simulink library "SUB_PLANT_Chassis"  (R2018a)
settings: Solver=VariableStepAuto  StartTime=0.0  StopTime=10.0  RelTol=1e-3
values from neighbouring files (symbols this model uses):
  Cf = 120000    [SUB_PLANT_LateralDynamics_CAL.mat]
  Cr = 240000    [SUB_PLANT_LateralDynamics_CAL.mat]
  GLB_FIXED_STEP_SIZE_CPV = ptc_matlab_lib.PTC_MBDS_Parameter('Value', 0.01,  	'Description', 'Global Fixed Step Size (Fundamental Sample Time)',  	'Unit', 's',  	'CoderInfo.StorageClass', 'Custom',  	'CoderInfo.CustomStorageClass', 'Const')    [GLB_CONST.m]
  heading_0 = 5.2    [SUB_PLANT_LateralDynamics_CAL.mat]
  Iz = 10000    [SUB_PLANT_LateralDynamics_CAL.mat]
  lf = 2.5    [SUB_PLANT_LateralDynamics_CAL.mat]
  lr = 3.5    [SUB_PLANT_LateralDynamics_CAL.mat]
  Vx_0 = 1    [SUB_PLANT_LateralDynamics_CAL.mat]
undefined symbols (not defined in the file or in its folder): DiscIntNeverNeededParam, GLB_TRANS_LOSS_TRQ_GEAR_STEP_MPV, GLB_TRANS_LOSS_TRQ_SPD_STEP_MPV, GLB_TRANS_LOSS_TRQ_TABLE_DATA_MPV, GLB_TRANS_LOSS_TRQ_TRQ_STEP_MPV
libraries: PTC_MBDS_LIB x41, simulink x6
(part 1 of 2)
settings Model: Creator=Sundeep.Tuteja  LastModifiedBy=Haris.Ashraf

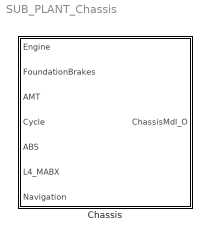
== system SUB_PLANT_Chassis ==
  Chassis : Subsystem

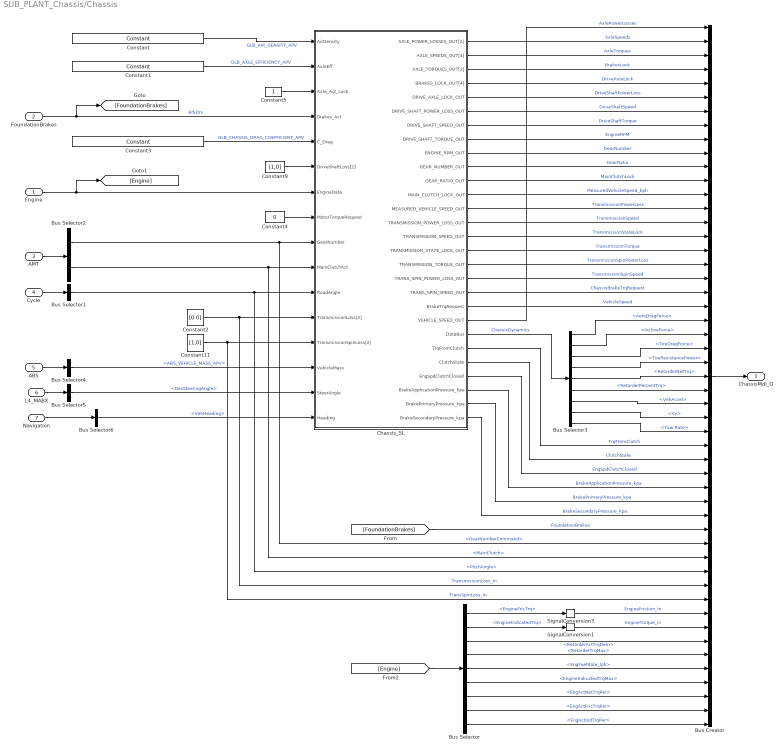
== system SUB_PLANT_Chassis/Chassis ==
  Engine : Inport
  FoundationBrakes : Inport  Port=2
  AMT : Inport  Port=3
  Cycle : Inport  Port=4
  ABS : Inport  Port=5
  L4_MABX : Inport  Port=6
  Navigation : Inport  Port=7
  Bus Creator : BusCreator  Inputs=51
  Bus Selector : BusSelector  OutputSignals=EngineFricTrq,EngineIndicatedTrq,RetarderActTrqDem,RetarderTrqMax,EngFuelRate_lph,EngineIndicatedTrqMax,EngActNetTrqPer,EngActFricTrqPer,EngActIndTrqPer
  Bus Selector1 : BusSelector  OutputSignals=PitchAngle
  Bus Selector2 : BusSelector  OutputSignals=ShiftControl.Internal.GearNumberCommand,ShiftControl.Internal.MainClutch
  Bus Selector3 : BusSelector  OutputSignals=AeroDragForce,InclineForce,TireDragForce,TireResistancePower,RetarderNetTrq,RetarderPercentTrq,VehAccel,Vy,Yaw Rate
  Bus Selector4 : BusSelector  OutputSignals=ABS_VEHICLE_MASS_APV
  Bus Selector5 : BusSelector  OutputSignals=10msTask.SteeringControl.DesSteeringAngle
  Bus Selector6 : BusSelector  OutputSignals=Navigation.VehHeading
  Chassis_SL : Subsystem
  Constant : PTC_MBDS_LIB/Extras/Sources/Constant  Value2=GLB_AIR_DENSITY_APV  PTC_MBDS_BlockVersion=5.41  PTC_BlockType=PTC_MBDS_Constant
      settings: SourceProductName=PACCAR Technical Center MBDS Library
      settings: AttributesFormatString=|
      | Value: 1.23696005344
      | Unit: 'kg/m^3'
  Constant1 : PTC_MBDS_LIB/Extras/Sources/Constant  Value2=GLB_AXLE_EFFICIENCY_APV  PTC_MBDS_BlockVersion=5.41  PTC_BlockType=PTC_MBDS_Constant
      settings: SourceProductName=PACCAR Technical Center MBDS Library
      settings: AttributesFormatString=|
      | Value: 0.980000019073
      | Unit: '1'
  Constant11 : Constant  Value=[1,0]
  Constant2 : Constant  Value=[0 0]
  Constant3 : PTC_MBDS_LIB/Extras/Sources/Constant  Value2=GLB_CHASSIS_DRAG_COEFFICIENT_APV  PTC_MBDS_BlockVersion=5.41  PTC_BlockType=PTC_MBDS_Constant
      settings: SourceProductName=PACCAR Technical Center MBDS Library
      settings: AttributesFormatString=|
      | Value: 0.65
      | Unit: '1'
  Constant4 : Constant  Value=0
  Constant5 : Constant
  Constant9 : Constant  Value=[1,0]
  SignalConversion1 : SignalConversion  ConversionOutput=Contiguous copy  OverrideOpt=off
  SignalConversion3 : SignalConversion  ConversionOutput=Contiguous copy  OverrideOpt=off
  ChassisMdl_O : Outport
  wires:
  Bus Selector6/1 -> Chassis_SL/16(Heading)  "<VehHeading>"
  Navigation/1 -> Bus Selector6/1
  Chassis_SL/25(EngSpdClutchClosed) -> Bus Creator/33  "EngSpdClutchClosed"
  Chassis_SL/24(ClutchState) -> Bus Creator/32  "ClutchState"
  Chassis_SL/23(TrqFromClutch) -> Bus Creator/31  "TrqFromClutch"
  Bus Selector2/1 -> Chassis_SL/9(GearNumber), Bus Creator/38  "<GearNumberCommand>"
  Chassis_SL/5(DRIVE_AXLE_LOCK_OUT) -> Bus Creator/5  "DriveAxleLock"
  Chassis_SL/11(GEAR_RATIO_OUT) -> Bus Creator/11  "GearRatio"
  Chassis_SL/3(AXLE_TORQUES_OUT[2]) -> Bus Creator/3  "AxleTorques"
  Chassis_SL/19(TRANS_SPIN_SPEED_OUT) -> Bus Creator/19  "TransmissionSpinSpeed"
  Chassis_SL/7(DRIVE_SHAFT_SPEED_OUT) -> Bus Creator/7  "DriveShaftSpeed"
  Chassis_SL/4(BRAKES_LOCK_OUT[4]) -> Bus Creator/4  "BrakesLock"
  Chassis_SL/18(TRANS_SPIN_POWER_LOSS_OUT) -> Bus Creator/18  "TransmissionSpinPowerLoss"
  Chassis_SL/6(DRIVE_SHAFT_POWER_LOSS_OUT) -> Bus Creator/6  "DrIveShaftPowerLoss"
  Chassis_SL/20(BrakeTrqRequest) -> Bus Creator/20  "ChassisBrakeTrqRequest"
  Chassis_SL/8(DRIVE_SHAFT_TORQUE_OUT) -> Bus Creator/8  "DriveShaftTorque"
  Chassis_SL/14(TRANSMISSION_POWER_LOSS_OUT) -> Bus Creator/14  "TransmissionPowerLoss"
  Constant1/1 -> Chassis_SL/2(AxleEff)  "GLB_AXLE_EFFICIENCY_APV"
  Constant5/1 -> Chassis_SL/3(Axle_Act_Lock)
  Constant3/1 -> Chassis_SL/5(C_Drag)  "GLB_CHASSIS_DRAG_COEFFICIENT_APV"
  Constant9/1 -> Chassis_SL/6(DriveShaftLoss[2])
  Constant11/1 -> Chassis_SL/13(TransmissionSpinLoss[2]), Bus Creator/42  "TransSpinLoss_In"
  Constant2/1 -> Chassis_SL/12(TransmissionLoss[2]), Bus Creator/41  "TransmisisonLoss_In"
  Bus Selector2/2 -> Bus Creator/39, Chassis_SL/10(MainClutchAct)  "<MainClutch>"
  Bus Creator/1 -> ChassisMdl_O/1
  Chassis_SL/1(AXLE_POWER_LOSSES_OUT[2]) -> Bus Creator/1  "AxlePowerLosses"
  Chassis_SL/9(ENGINE_RPM_OUT) -> Bus Creator/9  "EngineRPM"
  Chassis_SL/10(GEAR_NUMBER_OUT) -> Bus Creator/10  "GearNumber"
  Chassis_SL/12(MAIN_CLUTCH_LOCK_OUT) -> Bus Creator/12  "MainClutchLock"
  Chassis_SL/13(MEASURED_VEHICLE_SPEED_OUT) -> Bus Creator/13  "MeasuredVehicleSpeed_kph"
  Chassis_SL/16(TRANSMISSION_STATE_LOCK_OUT) -> Bus Creator/16  "TransmissionStateLock"
  Chassis_SL/17(TRANSMISSION_TORQUE_OUT) -> Bus Creator/17  "TransmissionTorque"
  Cycle/1 -> Bus Selector1/1
  Bus Selector1/1 -> Bus Creator/40, Chassis_SL/11(RoadAngle)  "<PitchAngle>"
  AMT/1 -> Bus Selector2/1
  FoundationBrakes/1 -> [FoundationBrakes], Chassis_SL/4(Brakes_Act)  "BrkDrv"
  [FoundationBrakes] -> Bus Creator/37  "FoundationBrakes"
  Bus Selector/7 -> Bus Creator/49  "<EngActNetTrqPer>"
  Bus Selector/8 -> Bus Creator/50  "<EngActFricTrqPer>"
  Chassis_SL/2(AXLE_SPEEDS_OUT[4]) -> Bus Creator/2  "AxleSpeeds"
  Chassis_SL/22(DataBus) -> Bus Selector3/1  "ChassisDynamics"
  Bus Selector3/1 -> Bus Creator/22  "<AeroDragForce>"
  Bus Selector3/2 -> Bus Creator/23  "<InclineForce>"
  Bus Selector3/4 -> Bus Creator/25  "<TireResistancePower>"
  Bus Selector3/5 -> Bus Creator/26  "<RetarderNetTrq>"
  Engine/1 -> [Engine], Chassis_SL/7(EngineData)
  [Engine] -> Bus Selector/1
  Bus Selector/1 -> SignalConversion3/1  "<EngineFricTrq>"
  Bus Selector/2 -> SignalConversion1/1  "<EngineIndicatedTrq>"
  Bus Selector3/6 -> Bus Creator/27  "<RetarderPercentTrq>"
  Bus Selector/3 -> Bus Creator/45  "<RetarderActTrqDem>"
  Bus Selector/4 -> Bus Creator/46  "<RetarderTrqMax>"
  Bus Selector3/7 -> Bus Creator/28  "<VehAccel>"
  Bus Selector/5 -> Bus Creator/47  "<EngFuelRate_lph>"
  Bus Selector3/3 -> Bus Creator/24  "<TireDragForce>"
  Bus Selector/6 -> Bus Creator/48  "<EngineIndicatedTrqMax>"
  Constant/1 -> Chassis_SL/1(AirDensity)  "GLB_AIR_DENSITY_APV"
  ABS/1 -> Bus Selector4/1
  Bus Selector4/1 -> Chassis_SL/14(VehicleMass)  "<ABS_VEHICLE_MASS_APV>"
  Chassis_SL/15(TRANSMISSION_SPEED_OUT) -> Bus Creator/15  "TransmissionSpeed"
  Chassis_SL/21(VEHICLE_SPEED_OUT) -> Bus Creator/21  "VehicleSpeed"
  Bus Selector/9 -> Bus Creator/51  "<EngActIndTrqPer>"
  SignalConversion3/1 -> Bus Creator/43  "EngineFriction_In"
  SignalConversion1/1 -> Bus Creator/44  "EngineTorque_in"
  Constant4/1 -> Chassis_SL/8(MotorTorqueRequest)
  Chassis_SL/26(BrakeApplicationPressure_kpa) -> Bus Creator/34  "BrakeApplicationPressure_kpa"
  Chassis_SL/27(BrakePrimaryPressure_kpa) -> Bus Creator/35  "BrakePrimaryPressure_kpa"
  Chassis_SL/28(BrakeSecondaryPressure_kpa) -> Bus Creator/36  "BrakeSecondaryPressure_kpa"
  Bus Selector3/8 -> Bus Creator/29  "<Vy>"
  Bus Selector3/9 -> Bus Creator/30  "<Yaw Rate>"
  L4_MABX/1 -> Bus Selector5/1
  Bus Selector5/1 -> Chassis_SL/15(SteerAngle)  "<DesSteeringAngle>"

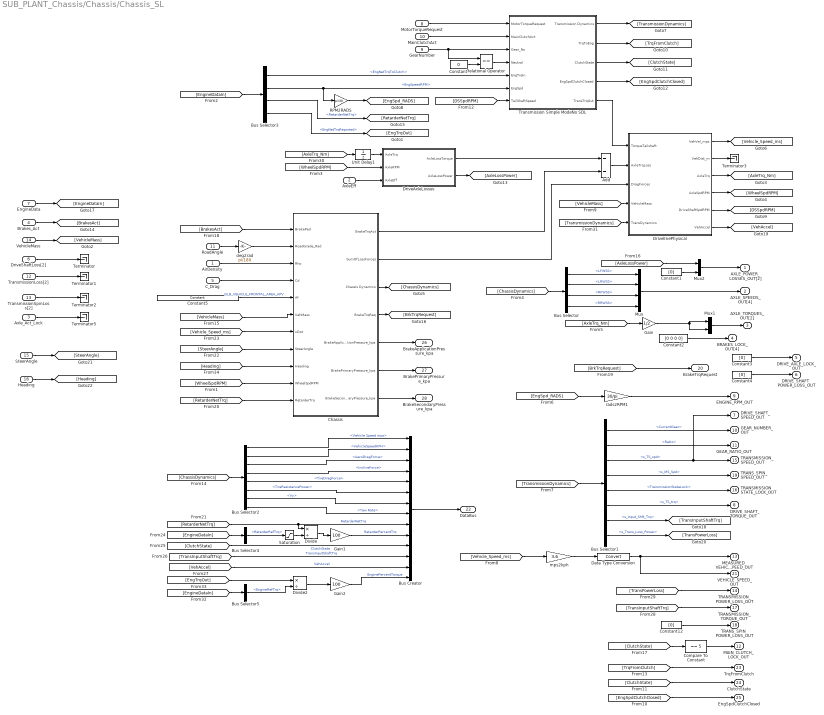
== system SUB_PLANT_Chassis/Chassis/Chassis_SL ==
  AirDensity : Inport
  AxleEff : Inport  Port=2
  Axle_Act_Lock : Inport  Port=3
  Brakes_Act : Inport  Port=4
  C_Drag : Inport  Port=5
  DriveShaftLoss[2] : Inport  Port=6
  EngineData : Inport  Port=7
  MotorTorqueRequest : Inport  Port=8
  GearNumber : Inport  Port=9
  MainClutchAct : Inport  Port=10
  RoadAngle : Inport  Port=11
  TransmissionLoss[2] : Inport  Port=12
  TransmissionSpinLoss[2] : Inport  Port=13
  VehicleMass : Inport  Port=14
  SteerAngle : Inport  Port=15
  Heading : Inport  Port=16
  Add : Sum  Inputs=--
  Bus Creator : BusCreator  Inputs=14
  Bus Selector : BusSelector  OutputSignals=Wheel Speed Sensors.LFWSS,Wheel Speed Sensors.LRWSS,Wheel Speed Sensors.RFWSS,Wheel Speed Sensors.RRWSS
  Bus Selector1 : BusSelector  OutputSignals=Gears_bus.CurrentGear,Gears_bus.Ratio,Gears_bus.s_TS_spd,Gears_bus.s_MS_Spd,MainClutch_bus.TransmissionStateLock,Gears_bus.s_TS_trq,s_Input_Shft_Trq,Gears_bus.s_Trans_Loss_Power
  Bus Selector2 : BusSelector  OutputSignals=Vehicle Speed mps,VehicleSpeedKPH,LongitudnalDynamics.AeroDragForce,LongitudnalDynamics.InclineForce,LongitudnalDynamics.TireDragForce,TireResistancePower,LateralDynamics.Vy,LateralDynamics.Yaw Rate
  Bus Selector3 : BusSelector  OutputSignals=EngNetTrqToClutch,EngSpeedRPM,RetarderNetTrq,EngNetTrqReported
  Bus Selector4 : BusSelector  OutputSignals=RetarderRefTrq
  Bus Selector5 : BusSelector  OutputSignals=EngineRefTrq
  Chassis : Subsystem
  Compare To Constant : simulink/Logic and Bit Operations/Compare To Constant  relop===  const=5  OutDataTypeStr=boolean
  Constant : Constant  Value=0
  Constant{1,3..4,12} (4 alike) : Constant  Value=[0]
  Constant2 : Constant  Value=[0 0 0 0]
  Constant5 : PTC_MBDS_LIB/Extras/Sources/Constant  Value2=GLB_VEHICLE_FRONTAL_AREA_APV  PTC_MBDS_BlockVersion=5.41  PTC_BlockType=PTC_MBDS_Constant
      settings: SourceProductName=PACCAR Technical Center MBDS Library
      settings: AttributesFormatString=|
      | Value: 10.38
      | Unit: 'm^2'
  Data Type Conversion : DataTypeConversion  SaturateOnIntegerOverflow=on
  Divide : Product  Inputs=*/
  Divide2 : Product  Inputs=*/
  DriveAxleLosses : Subsystem
  DrivelInePhysical : Subsystem
  Gain : Gain  Gain=1/2
  Gain1 : Gain  Gain=100
  Gain2 : Gain  Gain=100
  Mux : Mux
  Mux1 : Mux  Inputs=2
  Mux2 : Mux  Inputs=2
  RPM2RADS : Gain  Gain=pi/30
  Relational Operator : RelationalOperator  Operator===  OutDataTypeStr=boolean  RndMeth=Nearest
  Saturation : Saturate  UpperLimit=inf  LowerLimit=1
  Terminator{,1..3,5} (5 alike) : Terminator
      Terminator3 settings: InitFcn=|
      | try
      |    MBDS_BlockCallback('Update', gcb);
      | end
  Transmission Simple ModeNo SDL : Subsystem
  Unit Delay1 : UnitDelay  SampleTime=-1
  deg2rad : Gain  Gain=pi/180
  mps2kph : Gain  Gain=3.6
  rads2RPM1 : Gain  Gain=30/pi
  AXLE_POWER_LOSSES_OUT[2] : Outport
  AXLE_SPEEDS_OUT[4] : Outport  Port=2
  AXLE_TORQUES_OUT[2] : Outport  Port=3
  BRAKES_LOCK_OUT[4] : Outport  Port=4
  DRIVE_AXLE_LOCK_OUT : Outport  Port=5
  DRIVE_SHAFT_POWER_LOSS_OUT : Outport  Port=6
  DRIVE_SHAFT_SPEED_OUT : Outport  Port=7
  DRIVE_SHAFT_TORQUE_OUT : Outport  Port=8
  ENGINE_RPM_OUT : Outport  Port=9
  GEAR_NUMBER_OUT : Outport  Port=10
  GEAR_RATIO_OUT : Outport  Port=11
  MAIN_CLUTCH_LOCK_OUT : Outport  Port=12
  MEASURED_VEHICLE_SPEED_OUT : Outport  Port=13
  TRANSMISSION_POWER_LOSS_OUT : Outport  Port=14
  TRANSMISSION_SPEED_OUT : Outport  Port=15
  TRANSMISSION_STATE_LOCK_OUT : Outport  Port=16
  TRANSMISSION_TORQUE_OUT : Outport  Port=17
  TRANS_SPIN_POWER_LOSS_OUT : Outport  Port=18
  TRANS_SPIN_SPEED_OUT : Outport  Port=19
  BrakeTrqRequest : Outport  Port=20
  VEHICLE_SPEED_OUT : Outport  Port=21
  DataBus : Outport  Port=22
  TrqFromClutch : Outport  Port=23
  ClutchState : Outport  Port=24
  EngSpdClutchClosed : Outport  Port=25
  BrakeApplicationPressure_kpa : Outport  Port=26
  BrakePrimaryPressure_kpa : Outport  Port=27
  BrakeSecondaryPressure_kpa : Outport  Port=28
  wires:
  MotorTorqueRequest/1 -> Transmission Simple ModeNo SDL/1(MotorTorqueRequest)
  Bus Selector3/3 -> [RetarderNetTrq]  "<RetarderNetTrq>"
  Bus Selector3/2 -> Transmission Simple ModeNo SDL/6(EngSpd), RPM2RADS/1  "<EngSpeedRPM>"
  [EngineDataIn] -> Bus Selector3/1
  AirDensity/1 -> Chassis/3(Rho)
  C_Drag/1 -> Chassis/4(Cd)
  Constant5/1 -> Chassis/5(Af)  "GLB_VEHICLE_FRONTAL_AREA_APV"
  RoadAngle/1 -> deg2rad/1
  deg2rad/1 -> Chassis/2(RoadGrade_Rad)
  MainClutchAct/1 -> Transmission Simple ModeNo SDL/2(MainClutchAct)
  GearNumber/1 -> Relational Operator/1, Transmission Simple ModeNo SDL/3(Gear_No)
  Relational Operator/1 -> Transmission Simple ModeNo SDL/4(Neutral)
  Constant/1 -> Relational Operator/2
  Chassis/2(SumOfLossForces) -> DrivelInePhysical/3(DragForces)
  [BrakesAct] -> Chassis/1(BrakePed)
  [Vehicle_Speed_ms] -> Chassis/7(xDot)
  DrivelInePhysical/2(VehDist_m) -> Terminator3/1
  DriveAxleLosses/1(AxleLossTorque) -> Add/1
  Chassis/1(BrakeTrqAct) -> Add/2
  Add/1 -> DrivelInePhysical/2(AxleTrqLoss)
  DrivelInePhysical/3(AxleTrq) -> [AxleTrq_Nm]
  [AxleTrq_Nm] -> Unit Delay1/1
  AxleEff/1 -> DriveAxleLosses/3(AxleEff)
  [WheelSpdRPM] -> DriveAxleLosses/2(AxleRPM)
  DriveShaftLoss[2]/1 -> Terminator/1
  TransmissionLoss[2]/1 -> Terminator1/1
  TransmissionSpinLoss[2]/1 -> Terminator2/1
  Axle_Act_Lock/1 -> Terminator5/1
  Chassis/3(Chassis Dynamics) -> [ChassisDynamics]
  Transmission Simple ModeNo SDL/1(Transmission Dynamics) -> [TransmissionDynamics]
  [ChassisDynamics] -> Bus Selector/1
  Mux2/1 -> AXLE_POWER_LOSSES_OUT[2]/1
  Constant2/1 -> BRAKES_LOCK_OUT[4]/1
  Mux/1 -> AXLE_SPEEDS_OUT[4]/1
  Mux1/1 -> AXLE_TORQUES_OUT[2]/1
  Constant3/1 -> DRIVE_AXLE_LOCK_OUT/1
  Constant4/1 -> DRIVE_SHAFT_POWER_LOSS_OUT/1
  Bus Selector1/6 -> DRIVE_SHAFT_TORQUE_OUT/1  "<s_TS_trq>"
  [AxleTrq_Nm] -> Gain/1
  Gain/1 -> Mux1/2, Mux1/1
  [EngSpd_RADS] -> rads2RPM1/1
  rads2RPM1/1 -> ENGINE_RPM_OUT/1
  [TransmissionDynamics] -> Bus Selector1/1
  Bus Selector1/1 -> GEAR_NUMBER_OUT/1  "<CurrentGear>"
  Bus Selector1/2 -> GEAR_RATIO_OUT/1  "<Ratio>"
  Compare To Constant/1 -> MAIN_CLUTCH_LOCK_OUT/1
  [Vehicle_Speed_ms] -> mps2kph/1
  mps2kph/1 -> Data Type Conversion/1
  [TransPowerLoss] -> TRANSMISSION_POWER_LOSS_OUT/1
  Bus Selector1/5 -> TRANSMISSION_STATE_LOCK_OUT/1  "<TransmissionStateLock>"
  [TransInputShaftTrq] -> TRANSMISSION_TORQUE_OUT/1
  Constant12/1 -> TRANS_SPIN_POWER_LOSS_OUT/1
  Bus Selector1/4 -> TRANS_SPIN_SPEED_OUT/1  "<s_MS_Spd>"
  [BrkTrqRequest] -> BrakeTrqRequest/1
  Bus Selector1/3 -> TRANSMISSION_SPEED_OUT/1, DRIVE_SHAFT_SPEED_OUT/1  "<s_TS_spd>"
  DrivelInePhysical/4(AxleSpdRPM) -> [WheelSpdRPM]
  [WheelSpdRPM] -> Chassis/10(WheelSpdRPM)
  VehicleMass/1 -> [VehicleMass]
  [VehicleMass] -> DrivelInePhysical/4(VehicleMass)
  DrivelInePhysical/5(DriveShaftSpdRPM) -> [DSSpdRPM]
  [DSSpdRPM] -> Transmission Simple ModeNo SDL/7(TailShaftSpeed)
  Transmission Simple ModeNo SDL/2(TrqToEng) -> [TrqFromClutch]
  Transmission Simple ModeNo SDL/3(ClutchState) -> [ClutchState]
  [ClutchState] -> ClutchState/1
  [TrqFromClutch] -> TrqFromClutch/1
  Bus Selector3/1 -> Transmission Simple ModeNo SDL/5(EngTrqIn)  "<EngNetTrqToClutch>"
  Transmission Simple ModeNo SDL/4(EngSpdClutchClosed) -> [EngSpdClutchClosed]
  [EngSpdClutchClosed] -> EngSpdClutchClosed/1
  Transmission Simple ModeNo SDL/5(TransTrqOut) -> DrivelInePhysical/1(TorqueTailshaft)
  RPM2RADS/1 -> [EngSpd_RADS]
  [ChassisDynamics] -> Bus Selector2/1
  [VehicleMass] -> Chassis/6(VehMass)
  DriveAxleLosses/2(AxleLossPower) -> [AxleLossPower]
  [AxleLossPower] -> Mux2/1
  Constant1/1 -> Mux2/2
  [ClutchState] -> Compare To Constant/1
  Brakes_Act/1 -> [BrakesAct]
  Bus Selector3/4 -> [EngTrqOut]  "<EngNetTrqReported>"
  Chassis/4(BrakeTrqReq) -> [BrkTrqRequest]
  [RetarderNetTrq] -> Chassis/11(RetarderTrq)
  Bus Creator/1 -> DataBus/1
  [RetarderNetTrq] -> Bus Creator/9, Divide/1  "RetarderNetTrq"
  Bus Selector2/1 -> Bus Creator/1  "<Vehicle Speed mps>"
  Bus Selector2/2 -> Bus Creator/2  "<VehicleSpeedKPH>"
  Bus Selector2/3 -> Bus Creator/3  "<AeroDragForce>"
  Bus Selector2/4 -> Bus Creator/4  "<InclineForce>"
  Bus Selector2/6 -> Bus Creator/6  "<TireResistancePower>"
  EngineData/1 -> [EngineDataIn]
  [EngineDataIn] -> Bus Selector4/1
  Bus Selector4/1 -> Saturation/1  "<RetarderRefTrq>"
  Divide/1 -> Gain1/1
  Gain1/1 -> Bus Creator/10  "RetarderPercentTrq"
  [ClutchState] -> Bus Creator/11  "ClutchState"
  Bus Selector1/7 -> [TransInputShaftTrq]  "<s_Input_Shft_Trq>"
  [TransInputShaftTrq] -> Bus Creator/12  "TransInputShaftTrq"
  DrivelInePhysical/6(VehAccel) -> [VehAccel]
  [VehAccel] -> Bus Creator/13  "VehAccel"
  Saturation/1 -> Divide/2
  Bus Selector2/5 -> Bus Creator/5  "<TireDragForce>"
  Bus Selector1/8 -> [TransPowerLoss]  "<s_Trans_Loss_Power>"
  [TransmissionDynamics] -> DrivelInePhysical/5(TransDynamics)
  Unit Delay1/1 -> DriveAxleLosses/1(AxleTrq)
  Data Type Conversion/1 -> VEHICLE_SPEED_OUT/1, MEASURED_VEHICLE_SPEED_OUT/1
  Bus Selector/1 -> Mux/1  "<LFWSS>"
  Bus Selector/2 -> Mux/2  "<LRWSS>"
  Bus Selector/3 -> Mux/3  "<RFWSS>"
  Bus Selector/4 -> Mux/4  "<RRWSS>"
  [EngineDataIn] -> Bus Selector5/1
  Bus Selector5/1 -> Divide2/2  "<EngineRefTrq>"
  [EngTrqOut] -> Divide2/1
  Divide2/1 -> Gain2/1
  Gain2/1 -> Bus Creator/14  "EnginePercentTorque"
  Chassis/5(BrakeApplicationPressure_kpa) -> BrakeApplicationPressure_kpa/1
  Chassis/6(BrakePrimaryPressure_kpa) -> BrakePrimaryPressure_kpa/1
  Chassis/7(BrakeSecondaryPressure_kpa) -> BrakeSecondaryPressure_kpa/1
  SteerAngle/1 -> [SteerAngle]
  [SteerAngle] -> Chassis/8(SteerAngle)
  Bus Selector2/7 -> Bus Creator/7  "<Vy>"
  Bus Selector2/8 -> Bus Creator/8  "<Yaw Rate>"
  [Heading] -> Chassis/9(Heading)
  Heading/1 -> [Heading]
  DrivelInePhysical/1(VehVel_mps) -> [Vehicle_Speed_ms]

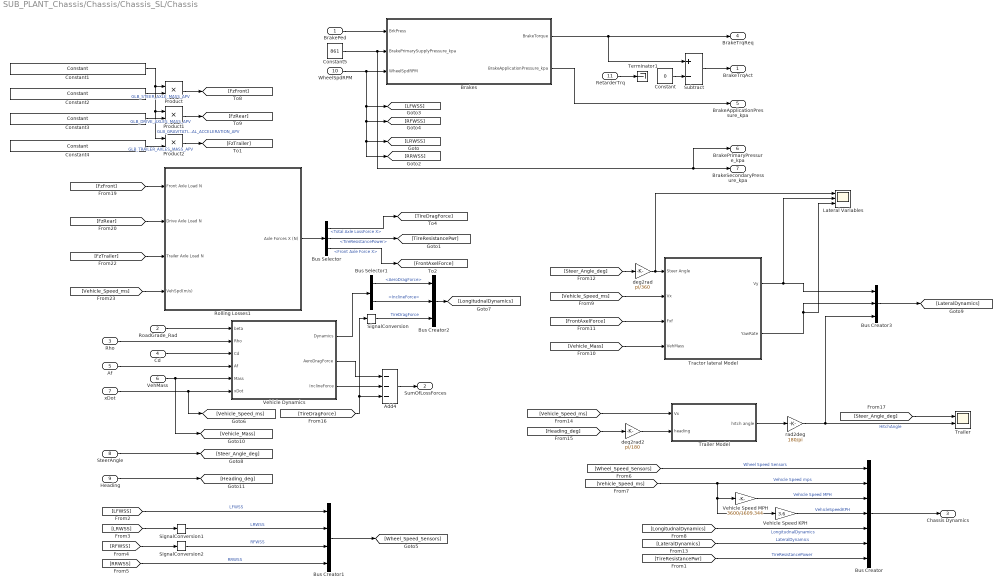
== system SUB_PLANT_Chassis/Chassis/Chassis_SL/Chassis ==
  BrakePed : Inport
  RoadGrade_Rad : Inport  Port=2
  Rho : Inport  Port=3
  Cd : Inport  Port=4
  Af : Inport  Port=5
  VehMass : Inport  Port=6
  xDot : Inport  Port=7
  SteerAngle : Inport  Port=8
  Heading : Inport  Port=9
  WheelSpdRPM : Inport  Port=10
  RetarderTrq : Inport  Port=11
  Add4 : Sum  Inputs=---
  Brakes : Subsystem
  Bus Creator : BusCreator  Inputs=7
  Bus Creator1 : BusCreator  Inputs=4
  Bus Creator2 : BusCreator  Inputs=3
  Bus Creator3 : BusCreator  Inputs=3
  Bus Selector : BusSelector  OutputSignals=Total Axle LossForce X,TireResistancePower,Front Axle Force X
  Bus Selector1 : BusSelector  OutputSignals=AeroDragForce,InclineForce
  Constant : Constant  Value=0
  Constant1 : PTC_MBDS_LIB/Extras/Sources/Constant  Value2=GLB_GRAVITATIONAL_ACCELERATION_APV  PTC_MBDS_BlockVersion=5.41  PTC_BlockType=PTC_MBDS_Constant
      settings: SourceProductName=PACCAR Technical Center MBDS Library
      settings: AttributesFormatString=|
      | Value: 9.80665016174
      | Unit: 'm/s^2'
  Constant2 : PTC_MBDS_LIB/Extras/Sources/Constant  Value2=GLB_STEER_AXLE_MASS_APV  PTC_MBDS_BlockVersion=5.41  PTC_BlockType=PTC_MBDS_Constant
      settings: SourceProductName=PACCAR Technical Center MBDS Library
      settings: AttributesFormatString=|
      | Value: 5261
      | Unit: 'kg'
  Constant3 : PTC_MBDS_LIB/Extras/Sources/Constant  Value2=GLB_DRIVE_AXLES_MASS_APV  PTC_MBDS_BlockVersion=5.41  PTC_BlockType=PTC_MBDS_Constant
      settings: SourceProductName=PACCAR Technical Center MBDS Library
      settings: AttributesFormatString=|
      | Value: 11770
      | Unit: 'kg'
  Constant4 : PTC_MBDS_LIB/Extras/Sources/Constant  Value2=GLB_TRAILER_AXLES_MASS_APV  PTC_MBDS_BlockVersion=5.41  PTC_BlockType=PTC_MBDS_Constant
      settings: SourceProductName=PACCAR Technical Center MBDS Library
      settings: AttributesFormatString=|
      | Value: 12460
      | Unit: 'kg'
  Constant5 : Constant  Value=861
  Lateral Variables : Scope  NumInputPorts=3
  Product : Product  Inputs=**  OutDataTypeStr=Inherit: Inherit via back propagation  SaturateOnIntegerOverflow=on  InputSameDT=on
      settings: AttributesFormatString=Saturate: %<SaturateOnIntegerOverflow>
  Product1 : Product  Inputs=**  OutDataTypeStr=Inherit: Inherit via back propagation  SaturateOnIntegerOverflow=on  InputSameDT=on
      settings: AttributesFormatString=Saturate: %<SaturateOnIntegerOverflow>
  Product2 : Product  Inputs=**  OutDataTypeStr=Inherit: Inherit via back propagation  SaturateOnIntegerOverflow=on  InputSameDT=on
      settings: AttributesFormatString=Saturate: %<SaturateOnIntegerOverflow>
  Rolling Losses1 : Subsystem
  SignalConversion : SignalConversion  ConversionOutput=Contiguous copy  OverrideOpt=off
  SignalConversion1 : SignalConversion  ConversionOutput=Contiguous copy  OverrideOpt=off
  SignalConversion2 : SignalConversion  ConversionOutput=Contiguous copy  OverrideOpt=off
  Subtract : Sum  Inputs=+-
  Terminator1 : Terminator
  Tractor lateral Model : Subsystem
  Trailer : Scope  NumInputPorts=2
  Trailer Model : Subsystem
  Vehicle Dynamics : Subsystem
  Vehicle Speed KPH : Gain  Gain=3.6
  Vehicle Speed MPH : Gain  Gain=3600/1609.344
  deg2rad : Gain  Gain=pi/360
  "deg2rad2 " : Gain  Gain=pi/180
  rad2deg : Gain  Gain=180/pi
  BrakeTrqAct : Outport
  SumOfLossForces : Outport  Port=2
  Chassis Dynamics : Outport  Port=3
  BrakeTrqReq : Outport  Port=4
  BrakeApplicationPressure_kpa : Outport  Port=5
  BrakePrimaryPressure_kpa : Outport  Port=6
  BrakeSecondaryPressure_kpa : Outport  Port=7
  wires:
  [LongitudnalDynamics] -> Bus Creator/5  "LongitudnalDynamics"
  Vehicle Dynamics/1(Dynamics) -> Bus Selector1/1
  Product2/1 -> [FzTrailer]
  Constant2/1 -> Product/2  "GLB_STEER_AXLE_MASS_APV"
  Product1/1 -> [FzRear]
  Product/1 -> [FzFront]
  Bus Selector/1 -> [TireDragForce]  "<Total Axle LossForce X>"
  Rolling Losses1/1("Axle Forces X (N) ") -> Bus Selector/1
  [Vehicle_Speed_ms] -> Rolling Losses1/4(VehSpd(m/s))
  [FzFront] -> Rolling Losses1/1(Front Axle Load N)
  [FzRear] -> Rolling Losses1/2(Drive Axle Load N)
  [FzTrailer] -> Rolling Losses1/3(Trailer Axle Load N)
  Vehicle Speed KPH/1 -> Bus Creator/4  "VehicleSpeedKPH"
  RoadGrade_Rad/1 -> Vehicle Dynamics/1(beta)
  Bus Creator1/1 -> [Wheel_Speed_Sensors]
  [LFWSS] -> Bus Creator1/1  "LFWSS"
  [RFWSS] -> SignalConversion2/1
  [LRWSS] -> SignalConversion1/1
  [RRWSS] -> Bus Creator1/4  "RRWSS"
  [Wheel_Speed_Sensors] -> Bus Creator/1  "Wheel Speed Sensors"
  Bus Creator/1 -> Chassis Dynamics/1
  [Vehicle_Speed_ms] -> Vehicle Speed KPH/1, Vehicle Speed MPH/1, Bus Creator/2  "Vehicle Speed mps"
  Vehicle Speed MPH/1 -> Bus Creator/3  "Vehicle Speed MPH"
  Rho/1 -> Vehicle Dynamics/2(Rho)
  Cd/1 -> Vehicle Dynamics/3(Cd)
  Af/1 -> Vehicle Dynamics/4(Af)
  xDot/1 -> Vehicle Dynamics/6(xDot), [Vehicle_Speed_ms]
  [TireDragForce] -> SignalConversion/1, Add4/3
  Vehicle Dynamics/3(InclineForce) -> Add4/2
  Vehicle Dynamics/2(AeroDragForce) -> Add4/1
  Add4/1 -> SumOfLossForces/1
  BrakePed/1 -> Brakes/1(BrkPress)
  WheelSpdRPM/1 -> [LFWSS], [RFWSS], [LRWSS], [RRWSS], Brakes/3(WheelSpdRPM)
  Brakes/1(BrakeTorque) -> BrakeTrqReq/1, Subtract/1
  [TireResistancePwr] -> Bus Creator/7  "TireResistancePower"
  Bus Selector/2 -> [TireResistancePwr]  "<TireResistancePower>"
  RetarderTrq/1 -> Terminator1/1
  Subtract/1 -> BrakeTrqAct/1
  Constant/1 -> Subtract/2
  Bus Creator2/1 -> [LongitudnalDynamics]
  Bus Selector1/2 -> Bus Creator2/2  "<InclineForce>"
  Bus Selector1/1 -> Bus Creator2/1  "<AeroDragForce>"
  Constant3/1 -> Product1/2  "GLB_DRIVE_AXLES_MASS_APV"
  Constant4/1 -> Product2/2  "GLB_TRAILER_AXLES_MASS_APV"
  Constant1/1 -> Product2/1, Product1/1, Product/1  "GLB_GRAVITATIONAL_ACCELERATION_APV"
  SignalConversion/1 -> Bus Creator2/3  "TireDragForce"
  SignalConversion1/1 -> Bus Creator1/2  "LRWSS"
  SignalConversion2/1 -> Bus Creator1/3  "RFWSS"
  Brakes/2(BrakeApplicationPressure_kpa) -> BrakeApplicationPressure_kpa/1
  Constant5/1 -> BrakePrimaryPressure_kpa/1, BrakeSecondaryPressure_kpa/1, Brakes/2(BrakePrimarySupplyPressure_kpa)
  Tractor lateral Model/1(Vy) -> Lateral Variables/2, Bus Creator3/1
  Tractor lateral Model/2(YawRate) -> Lateral Variables/3, Bus Creator3/2
  [Vehicle_Mass] -> Tractor lateral Model/4(VehMass)
  Bus Creator3/1 -> [LateralDynamics]
  Bus Selector/3 -> [FrontAxelForce]  "<Front Axle Force X>"
  [FrontAxelForce] -> Tractor lateral Model/3(Fxf)
  SteerAngle/1 -> [Steer_Angle_deg]
  [Steer_Angle_deg] -> deg2rad/1
  deg2rad/1 -> Lateral Variables/1, Tractor lateral Model/1(Steer Angle)
  [LateralDynamics] -> Bus Creator/6  "LateralDynamics"
  VehMass/1 -> [Vehicle_Mass], Vehicle Dynamics/5(Mass)
  [Vehicle_Speed_ms] -> Tractor lateral Model/2(Vx)
  [Vehicle_Speed_ms] -> Trailer Model/1(Vx)
  Heading/1 -> [Heading_deg]
  "deg2rad2 "/1 -> Trailer Model/2(heading)
  [Heading_deg] -> "deg2rad2 "/1
  [Steer_Angle_deg] -> Trailer/1
  rad2deg/1 -> Trailer/2, Bus Creator3/3  "HitchAngle"
  Trailer Model/1(hitch angle) -> rad2deg/1

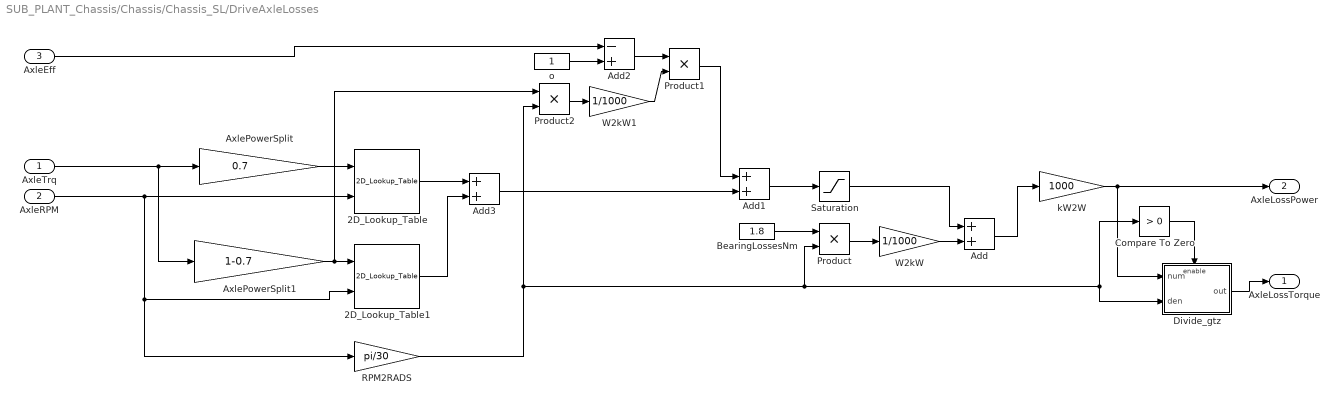
== system SUB_PLANT_Chassis/Chassis/Chassis_SL/DriveAxleLosses ==
  AxleTrq : Inport
  AxleRPM : Inport  Port=2
  AxleEff : Inport  Port=3
  2D_Lookup_Table : PTC_MBDS_LIB/Extras/Lookup Tables/2D_Lookup_Table  ParameterObjectName=GLB_AXLE_POWER_LOSS_DATA_MPV  InterpolationMethod=Linear  PTC_MBDS_BlockVersion=5.41  PTC_BlockType=PTC_MBDS_2D_Lookup_Table
      settings: SourceProductName=PACCAR Technical Center MBDS Library
      settings: AttributesFormatString=|
      | Row Axis: GLB_AXLE_POWER_LOSS_AXLETRQ_STEP_MPV (N*m)
      | Column Axis: GLB_AXLE_POWER_LOSS_AXLESPD_STEP_MPV (rpm)
      | Data Axis: GLB_AXLE_POWER_LOSS_DATA_MPV (kW)
      | Interpolation Method: Linear
  2D_Lookup_Table1 : PTC_MBDS_LIB/Extras/Lookup Tables/2D_Lookup_Table  ParameterObjectName=GLB_AXLE_POWER_LOSS_DATA_MPV  InterpolationMethod=Linear  PTC_MBDS_BlockVersion=5.41  PTC_BlockType=PTC_MBDS_2D_Lookup_Table
      settings: SourceProductName=PACCAR Technical Center MBDS Library
      settings: AttributesFormatString=|
      | Row Axis: GLB_AXLE_POWER_LOSS_AXLETRQ_STEP_MPV (N*m)
      | Column Axis: GLB_AXLE_POWER_LOSS_AXLESPD_STEP_MPV (rpm)
      | Data Axis: GLB_AXLE_POWER_LOSS_DATA_MPV (kW)
      | Interpolation Method: Linear
  Add : Sum
  Add1 : Sum
  Add2 : Sum  Inputs=-+
  Add3 : Sum
  AxlePowerSplit : Gain  Gain=0.7
  AxlePowerSplit1 : Gain  Gain=1-0.7
  BearingLossesNm : Constant  Value=1.8
  Compare To Zero : simulink/Logic and Bit Operations/Compare To Zero  relop=>  OutDataTypeStr=boolean
  Divide_gtz : Subsystem
  Product : Product  Inputs=**
  Product1 : Product  Inputs=**
  Product2 : Product  Inputs=**
  RPM2RADS : Gain  Gain=pi/30
  Saturation : Saturate  UpperLimit=Inf  LowerLimit=0
  W2kW : Gain  Gain=1/1000
  W2kW1 : Gain  Gain=1/1000
  kW2W : Gain  Gain=1000
  o : Constant
  AxleLossTorque : Outport
  AxleLossPower : Outport  Port=2
  wires:
  AxleRPM/1 -> 2D_Lookup_Table/2, 2D_Lookup_Table1/2, RPM2RADS/1
  Saturation/1 -> Add/1
  kW2W/1 -> AxleLossPower/1, Divide_gtz/1(num)
  AxleTrq/1 -> AxlePowerSplit/1, AxlePowerSplit1/1
  Add1/1 -> Saturation/1
  BearingLossesNm/1 -> Product/1
  Product/1 -> W2kW/1
  Add/1 -> kW2W/1
  W2kW/1 -> Add/2
  RPM2RADS/1 -> Product2/2, Product/2, Compare To Zero/1, Divide_gtz/2(den)
  Add2/1 -> Product1/1
  AxleEff/1 -> Add2/1
  Product1/1 -> Add1/1
  o/1 -> Add2/2
  Compare To Zero/1 -> Divide_gtz/Enable
  W2kW1/1 -> Product1/2
  Product2/1 -> W2kW1/1
  2D_Lookup_Table/1 -> Add3/1
  2D_Lookup_Table1/1 -> Add3/2
  AxlePowerSplit/1 -> 2D_Lookup_Table/1
  AxlePowerSplit1/1 -> 2D_Lookup_Table1/1, Product2/1
  Add3/1 -> Add1/2
  Divide_gtz/1(out) -> AxleLossTorque/1

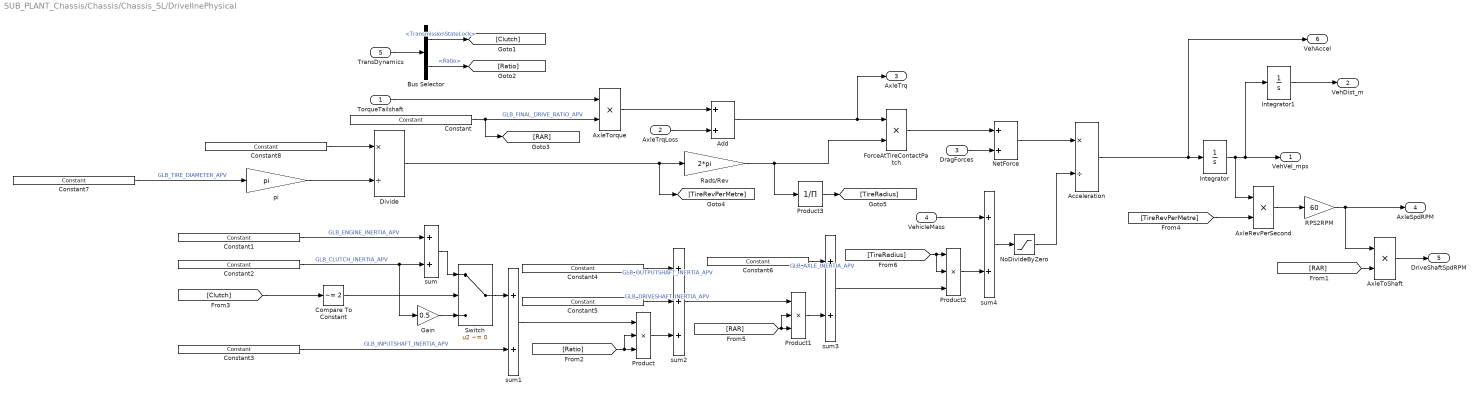
== system SUB_PLANT_Chassis/Chassis/Chassis_SL/DrivelInePhysical ==
  TorqueTailshaft : Inport
  AxleTrqLoss : Inport  Port=2
  DragForces : Inport  Port=3
  VehicleMass : Inport  Port=4
  TransDynamics : Inport  Port=5
  Acceleration : Product  Inputs=*/
  Add : Sum
  AxleRevPerSecond : Product
  AxleToShaft : Product
  AxleTorque : Product
  Bus Selector : BusSelector  OutputSignals=MainClutch_bus.TransmissionStateLock,Gears_bus.Ratio
  Compare To Constant : simulink/Logic and Bit Operations/Compare To Constant  relop=~=  const=2  OutDataTypeStr=boolean
  Constant : PTC_MBDS_LIB/Extras/Sources/Constant  Value2=GLB_FINAL_DRIVE_RATIO_APV  PTC_MBDS_BlockVersion=5.41  PTC_BlockType=PTC_MBDS_Constant
      settings: SourceProductName=PACCAR Technical Center MBDS Library
      settings: AttributesFormatString=|
      | Value: 2.79
      | Unit: '1'
  Constant1 : PTC_MBDS_LIB/Extras/Sources/Constant  Value2=GLB_ENGINE_INERTIA_APV  PTC_MBDS_BlockVersion=5.41  PTC_BlockType=PTC_MBDS_Constant
      settings: SourceProductName=PACCAR Technical Center MBDS Library
      settings: AttributesFormatString=|
      | Value: 3.7109375
      | Unit: 'kg*m^2'
  Constant2 : PTC_MBDS_LIB/Extras/Sources/Constant  Value2=GLB_CLUTCH_INERTIA_APV  PTC_MBDS_BlockVersion=5.41  PTC_BlockType=PTC_MBDS_Constant
      settings: SourceProductName=PACCAR Technical Center MBDS Library
      settings: AttributesFormatString=|
      | Value: 0.115966796875
      | Unit: 'kg*m^2'
  Constant3 : PTC_MBDS_LIB/Extras/Sources/Constant  Value2=GLB_INPUTSHAFT_INERTIA_APV  PTC_MBDS_BlockVersion=5.41  PTC_BlockType=PTC_MBDS_Constant
      settings: SourceProductName=PACCAR Technical Center MBDS Library
      settings: AttributesFormatString=|
      | Value: 0.015
      | Unit: 'kg*m^2'
  Constant4 : PTC_MBDS_LIB/Extras/Sources/Constant  Value2=GLB_OUTPUTSHAFT_INERTIA_APV  PTC_MBDS_BlockVersion=5.41  PTC_BlockType=PTC_MBDS_Constant
      settings: SourceProductName=PACCAR Technical Center MBDS Library
      settings: AttributesFormatString=|
      | Value: 0.03
      | Unit: 'kg*m^2'
  Constant5 : PTC_MBDS_LIB/Extras/Sources/Constant  Value2=GLB_DRIVESHAFT_INERTIA_APV  PTC_MBDS_BlockVersion=5.41  PTC_BlockType=PTC_MBDS_Constant
      settings: SourceProductName=PACCAR Technical Center MBDS Library
      settings: AttributesFormatString=|
      | Value: 0.001
      | Unit: 'kg*m^2'
  Constant6 : PTC_MBDS_LIB/Extras/Sources/Constant  Value2=GLB_AXLE_INERTIA_APV  PTC_MBDS_BlockVersion=5.41  PTC_BlockType=PTC_MBDS_Constant
      settings: SourceProductName=PACCAR Technical Center MBDS Library
      settings: AttributesFormatString=|
      | Value: 0.10000000149
      | Unit: 'kg*m^2'
  Constant7 : PTC_MBDS_LIB/Extras/Sources/Constant  Value2=GLB_TIRE_DIAMETER_APV  PTC_MBDS_BlockVersion=5.41  PTC_BlockType=PTC_MBDS_Constant
      settings: SourceProductName=PACCAR Technical Center MBDS Library
      settings: AttributesFormatString=|
      | Value: 1
      | Unit: 'm'
  Constant8 : PTC_MBDS_LIB/Extras/Sources/Constant  Value2=1  PTC_MBDS_BlockVersion=5.41  PTC_BlockType=PTC_MBDS_Constant
      settings: SourceProductName=PACCAR Technical Center MBDS Library
  Divide : Product  Inputs=*/  OutDataTypeStr=Inherit: Inherit via back propagation  SaturateOnIntegerOverflow=on  InputSameDT=on
      settings: AttributesFormatString=Saturate: %<SaturateOnIntegerOverflow>
  ForceAtTireContactPatch : Product
  Gain : Gain  Gain=0.5
  Integrator : Integrator  InitialCondition=Vx_0  LimitOutput=on  UpperSaturationLimit=1000  LowerSaturationLimit=0
  Integrator1 : Integrator  LimitOutput=on  LowerSaturationLimit=0
  NetForce : Sum
  NoDivideByZero : Saturate  UpperLimit=inf  LowerLimit=1
  Product : Product  Inputs=3
  Product1 : Product  Inputs=3
  Product2 : Product  Inputs=3
  Product3 : Product  Inputs=/
  RPS2RPM : Gain  Gain=60
  Rads/Rev : Gain  Gain=2*pi
  Switch : Switch  Criteria=u2 ~= 0
  pi : Gain  Gain=pi
  sum{,1,3..4} (4 alike) : Sum
  sum2 : Sum  Inputs=3
  VehVel_mps : Outport
  VehDist_m : Outport  Port=2
  AxleTrq : Outport  Port=3
  AxleSpdRPM : Outport  Port=4
  DriveShaftSpdRPM : Outport  Port=5
  VehAccel : Outport  Port=6
  wires:
  TorqueTailshaft/1 -> AxleTorque/1
  Constant/1 -> [RAR], AxleTorque/2  "GLB_FINAL_DRIVE_RATIO_APV"
  AxleTorque/1 -> Add/1
  Divide/1 -> [TireRevPerMetre], Rads/Rev/1
  Rads/Rev/1 -> Product3/1, ForceAtTireContactPatch/2
  AxleTrqLoss/1 -> Add/2
  Add/1 -> AxleTrq/1, ForceAtTireContactPatch/1
  ForceAtTireContactPatch/1 -> NetForce/1
  DragForces/1 -> NetForce/2
  NetForce/1 -> Acceleration/1
  NoDivideByZero/1 -> Acceleration/2
  Acceleration/1 -> VehAccel/1, Integrator/1
  Integrator/1 -> AxleRevPerSecond/1, Integrator1/1, VehVel_mps/1
  Integrator1/1 -> VehDist_m/1
  AxleRevPerSecond/1 -> RPS2RPM/1
  RPS2RPM/1 -> AxleToShaft/1, AxleSpdRPM/1
  AxleToShaft/1 -> DriveShaftSpdRPM/1
  TransDynamics/1 -> Bus Selector/1
  [Clutch] -> Compare To Constant/1
  Compare To Constant/1 -> Switch/2
  Constant1/1 -> sum/1  "GLB_ENGINE_INERTIA_APV"
  Constant2/1 -> Gain/1, sum/2  "GLB_CLUTCH_INERTIA_APV"
  Gain/1 -> Switch/3
  sum/1 -> Switch/1
  Bus Selector/1 -> [Clutch]  "<TransmissionStateLock>"
  Bus Selector/2 -> [Ratio]  "<Ratio>"
  [TireRevPerMetre] -> AxleRevPerSecond/2
  [RAR] -> AxleToShaft/2
  Constant3/1 -> sum1/2  "GLB_INPUTSHAFT_INERTIA_APV"
  Switch/1 -> sum1/1
  [Ratio] -> Product/2, Product/3
  sum1/1 -> Product/1
  Product/1 -> sum2/3
  Constant5/1 -> sum2/2  "GLB_DRIVESHAFT_INERTIA_APV"
  Constant4/1 -> sum2/1  "GLB_OUTPUTSHAFT_INERTIA_APV"
  [RAR] -> Product1/2, Product1/3
  sum2/1 -> Product1/1
  Constant6/1 -> sum3/1  "GLB_AXLE_INERTIA_APV"
  Product1/1 -> sum3/2
  Product2/1 -> sum4/2
  sum4/1 -> NoDivideByZero/1
  sum3/1 -> Product2/3
  [TireRadius] -> Product2/2, Product2/1
  Product3/1 -> [TireRadius]
  VehicleMass/1 -> sum4/1
  Constant7/1 -> pi/1  "GLB_TIRE_DIAMETER_APV"
  pi/1 -> Divide/2
  Constant8/1 -> Divide/1

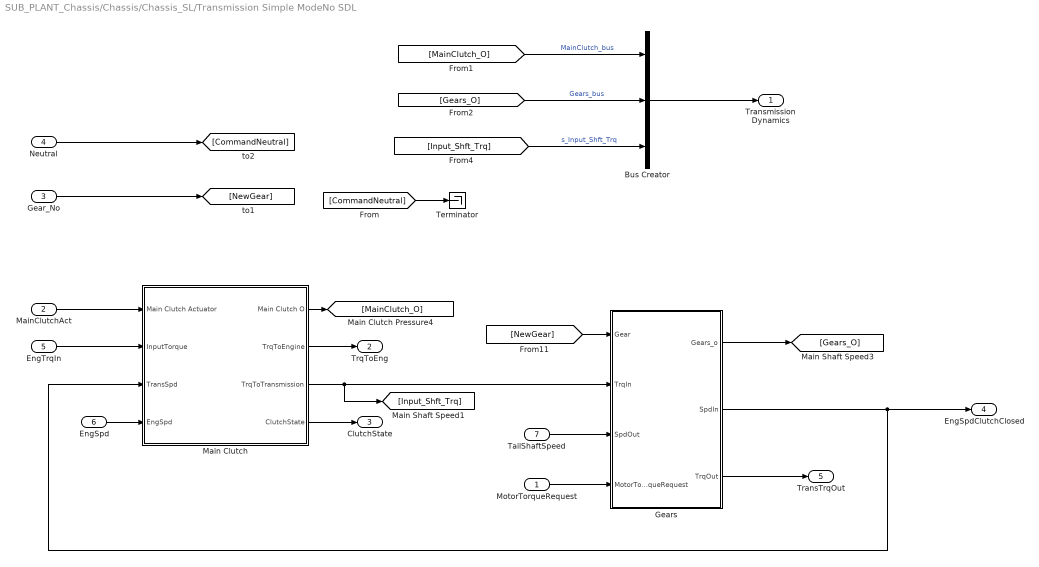
== system SUB_PLANT_Chassis/Chassis/Chassis_SL/Transmission Simple ModeNo SDL ==
  MotorTorqueRequest : Inport
  MainClutchAct : Inport  Port=2
  Gear_No : Inport  Port=3
  Neutral : Inport  Port=4
  EngTrqIn : Inport  Port=5
  EngSpd : Inport  Port=6
  TailShaftSpeed : Inport  Port=7
  Bus Creator : BusCreator  Inputs=3
  Gears : Subsystem
  Main Clutch : Subsystem
  Terminator : Terminator
      settings: InitFcn=|
      | try
      |    MBDS_BlockCallback('Update', gcb);
      | end
  Transmission Dynamics : Outport
  TrqToEng : Outport  Port=2
  ClutchState : Outport  Port=3
  EngSpdClutchClosed : Outport  Port=4
  TransTrqOut : Outport  Port=5
  wires:
  MotorTorqueRequest/1 -> Gears/4(MotorTorqueRequest)
  [Input_Shft_Trq] -> Bus Creator/3  "s_Input_Shft_Trq"
  [NewGear] -> Gears/1(Gear)
  Bus Creator/1 -> Transmission Dynamics/1
  Main Clutch/1(Main Clutch O) -> [MainClutch_O]
  [MainClutch_O] -> Bus Creator/1  "MainClutch_bus"
  [Gears_O] -> Bus Creator/2  "Gears_bus"
  Gear_No/1 -> [NewGear]
  Gears/1(Gears_o) -> [Gears_O]
  Main Clutch/3(TrqToTransmission) -> [Input_Shft_Trq], Gears/2(TrqIn)
  MainClutchAct/1 -> Main Clutch/1(Main Clutch Actuator)
  Neutral/1 -> [CommandNeutral]
  EngSpd/1 -> Main Clutch/4(EngSpd)
  Gears/2(SpdIn) -> Main Clutch/3(TransSpd), EngSpdClutchClosed/1
  EngTrqIn/1 -> Main Clutch/2(InputTorque)
  Main Clutch/4(ClutchState) -> ClutchState/1
  Main Clutch/2(TrqToEngine) -> TrqToEng/1
  Gears/3(TrqOut) -> TransTrqOut/1
  TailShaftSpeed/1 -> Gears/3(SpdOut)
  [CommandNeutral] -> Terminator/1

== system SUB_PLANT_Chassis/Chassis/Chassis_SL/Chassis/Brakes ==
  BrkPress : Inport
  BrakePrimarySupplyPressure_kpa : Inport  Port=2
  WheelSpdRPM : Inport  Port=3
  1-D Lookup Table : Lookup_n-D  NumberOfTableDimensions=1  BreakpointsForDimension1=[0 .1 1 10]  Table=[0 .1 .5 1]  ExtrapMethod=Clip  UseLastTableValue=on  RndMeth=Simplest  InputSameDT=on
  BrakeTorq Table : Lookup_n-D  NumberOfTableDimensions=1  BreakpointsForDimension1=[0:.1:1]  Table=[0 100 500 1000 2000 4000 8000 16000 20000 24000 50000]  RndMeth=Simplest  InputSameDT=on
  Gain : Gain  Gain=10
  NetBrakeTrq : Product  RndMeth=Zero
  Product : Product  RndMeth=Zero
  BrakeTorque : Outport
  BrakeApplicationPressure_kpa : Outport  Port=2
  wires:
  WheelSpdRPM/1 -> 1-D Lookup Table/1
  BrakeTorq Table/1 -> NetBrakeTrq/1
  BrkPress/1 -> BrakeTorq Table/1, Product/2
  1-D Lookup Table/1 -> NetBrakeTrq/2
  NetBrakeTrq/1 -> Gain/1
  Gain/1 -> BrakeTorque/1
  Product/1 -> BrakeApplicationPressure_kpa/1
  BrakePrimarySupplyPressure_kpa/1 -> Product/1

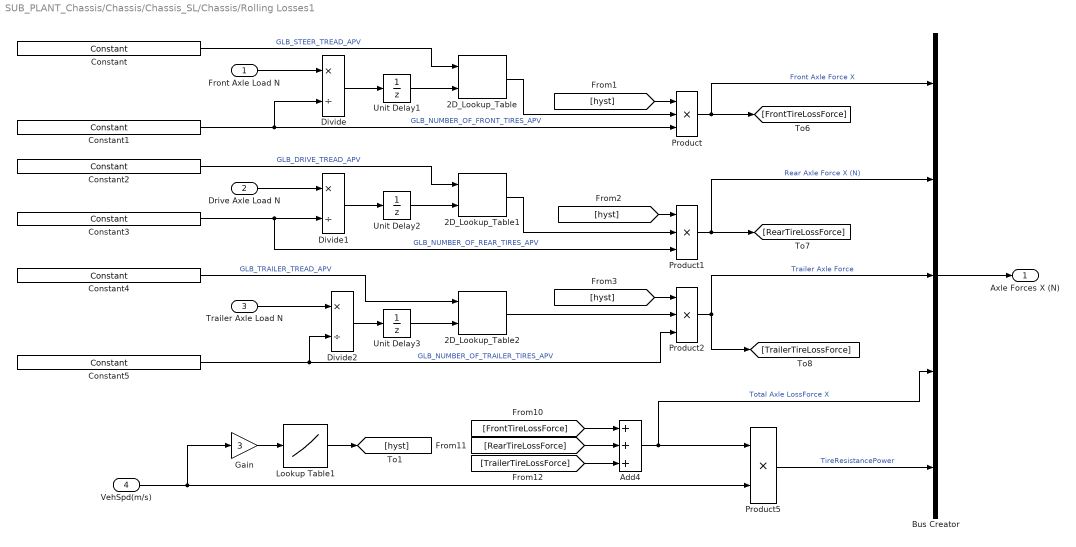
== system SUB_PLANT_Chassis/Chassis/Chassis_SL/Chassis/Rolling Losses1 ==
  Front Axle Load N : Inport
  Drive Axle Load N : Inport  Port=2
  Trailer Axle Load N : Inport  Port=3
  VehSpd(m/s) : Inport  Port=4
  2D_Lookup_Table : PTC_MBDS_LIB/Extras/Lookup Tables/2D_Lookup_Table  ParameterObjectName=GLB_STEER_TIRE_RRVSLOAD_RES_MPV  InterpolationMethod=Linear  PTC_MBDS_BlockVersion=5.41  PTC_BlockType=PTC_MBDS_2D_Lookup_Table
      settings: SourceProductName=PACCAR Technical Center MBDS Library
      settings: AttributesFormatString=|
      | Row Axis: GLB_STEER_TIRE_RRVSLOAD_TREAD_MPV (in/32)
      | Column Axis: GLB_STEER_TIRE_RRVSLOAD_LOAD_MPV (N)
      | Data Axis: GLB_STEER_TIRE_RRVSLOAD_RES_MPV (N)
      | Interpolation Method: Linear
  2D_Lookup_Table1 : PTC_MBDS_LIB/Extras/Lookup Tables/2D_Lookup_Table  ParameterObjectName=GLB_DRIVE_TIRE_RRVSLOAD_RES_MPV  InterpolationMethod=Linear  PTC_MBDS_BlockVersion=5.41  PTC_BlockType=PTC_MBDS_2D_Lookup_Table
      settings: SourceProductName=PACCAR Technical Center MBDS Library
      settings: AttributesFormatString=|
      | Row Axis: GLB_DRIVE_TIRE_RRVSLOAD_TREAD_MPV (in/32)
      | Column Axis: GLB_DRIVE_TIRE_RRVSLOAD_LOAD_MPV (N)
      | Data Axis: GLB_DRIVE_TIRE_RRVSLOAD_RES_MPV (N)
      | Interpolation Method: Linear
  2D_Lookup_Table2 : PTC_MBDS_LIB/Extras/Lookup Tables/2D_Lookup_Table  ParameterObjectName=GLB_TRAILER_TIRE_RRVSLOAD_RES_MPV  InterpolationMethod=Linear  PTC_MBDS_BlockVersion=5.41  PTC_BlockType=PTC_MBDS_2D_Lookup_Table
      settings: SourceProductName=PACCAR Technical Center MBDS Library
      settings: AttributesFormatString=|
      | Row Axis: GLB_TRAILER_TIRE_RRVSLOAD_TREAD_MPV (in/32)
      | Column Axis: GLB_TRAILER_TIRE_RRVSLOAD_LOAD_MPV (N)
      | Data Axis: GLB_TRAILER_TIRE_RRVSLOAD_RES_MPV (N)
      | Interpolation Method: Linear
  Add4 : Sum  Inputs=+++
  Bus Creator : BusCreator  Inputs=5
  Constant : PTC_MBDS_LIB/Extras/Sources/Constant  Value2=GLB_STEER_TREAD_APV  PTC_MBDS_BlockVersion=5.41  PTC_BlockType=PTC_MBDS_Constant
      settings: SourceProductName=PACCAR Technical Center MBDS Library
      settings: AttributesFormatString=|
      | Value: 24
      | Unit: 'in/32'
  Constant1 : PTC_MBDS_LIB/Extras/Sources/Constant  Value2=GLB_NUMBER_OF_FRONT_TIRES_APV  PTC_MBDS_BlockVersion=5.41  PTC_BlockType=PTC_MBDS_Constant
      settings: SourceProductName=PACCAR Technical Center MBDS Library
      settings: AttributesFormatString=|
      | Value: 2
      | Unit: '1'
  Constant2 : PTC_MBDS_LIB/Extras/Sources/Constant  Value2=GLB_DRIVE_TREAD_APV  PTC_MBDS_BlockVersion=5.41  PTC_BlockType=PTC_MBDS_Constant
      settings: SourceProductName=PACCAR Technical Center MBDS Library
      settings: AttributesFormatString=|
      | Value: 24
      | Unit: 'in/32'
  Constant3 : PTC_MBDS_LIB/Extras/Sources/Constant  Value2=GLB_NUMBER_OF_REAR_TIRES_APV  PTC_MBDS_BlockVersion=5.41  PTC_BlockType=PTC_MBDS_Constant
      settings: SourceProductName=PACCAR Technical Center MBDS Library
      settings: AttributesFormatString=|
      | Value: 8
      | Unit: '1'
  Constant4 : PTC_MBDS_LIB/Extras/Sources/Constant  Value2=GLB_TRAILER_TREAD_APV  PTC_MBDS_BlockVersion=5.41  PTC_BlockType=PTC_MBDS_Constant
      settings: SourceProductName=PACCAR Technical Center MBDS Library
      settings: AttributesFormatString=|
      | Value: 24
      | Unit: 'in/32'
  Constant5 : PTC_MBDS_LIB/Extras/Sources/Constant  Value2=GLB_NUMBER_OF_TRAILER_TIRES_APV  PTC_MBDS_BlockVersion=5.41  PTC_BlockType=PTC_MBDS_Constant
      settings: SourceProductName=PACCAR Technical Center MBDS Library
      settings: AttributesFormatString=|
      | Value: 8
      | Unit: '1'
  Divide : Product  Inputs=*/
  Divide1 : Product  Inputs=*/
  Divide2 : Product  Inputs=*/
  Gain : Gain  Gain=3
  Lookup Table1 : Lookup  InputValues=[-5:5]  Table=tanh([-5:5])  LookUpMeth=Interpolation-Use End Values
  Product : Product  Inputs=3  RndMeth=Zero
  Product1 : Product  Inputs=3  RndMeth=Zero
  Product2 : Product  Inputs=3  RndMeth=Zero
  Product5 : Product  RndMeth=Zero
  Unit Delay1 : UnitDelay  SampleTime=-1
  Unit Delay2 : UnitDelay  SampleTime=-1
  Unit Delay3 : UnitDelay  SampleTime=-1
  "Axle Forces X (N) " : Outport
  wires:
  Product5/1 -> Bus Creator/5  "TireResistancePower"
  [hyst] -> Product1/1
  [hyst] -> Product/1
  [TrailerTireLossForce] -> Add4/3
  [RearTireLossForce] -> Add4/2
  [FrontTireLossForce] -> Add4/1
  VehSpd(m/s)/1 -> Product5/2, Gain/1
  Add4/1 -> Product5/1, Bus Creator/4  "Total Axle LossForce X"
  Product2/1 -> [TrailerTireLossForce], Bus Creator/3  "Trailer Axle Force"
  Product/1 -> Bus Creator/1, [FrontTireLossForce]  "Front Axle Force X"
  [hyst] -> Product2/1
  2D_Lookup_Table2/1 -> Product2/2
  Lookup Table1/1 -> [hyst]
  Gain/1 -> Lookup Table1/1
  Bus Creator/1 -> "Axle Forces X (N) "/1
  2D_Lookup_Table1/1 -> Product1/2
  2D_Lookup_Table/1 -> Product/2
  Product1/1 -> Bus Creator/2, [RearTireLossForce]  "Rear Axle Force X (N)"
  Front Axle Load N/1 -> Divide/1
  Drive Axle Load N/1 -> Divide1/1
  Unit Delay1/1 -> 2D_Lookup_Table/2
  Unit Delay3/1 -> 2D_Lookup_Table2/2
  Constant4/1 -> 2D_Lookup_Table2/1  "GLB_TRAILER_TREAD_APV"
  Trailer Axle Load N/1 -> Divide2/1
  Divide/1 -> Unit Delay1/1
  Divide1/1 -> Unit Delay2/1
  Constant3/1 -> Product1/3, Divide1/2  "GLB_NUMBER_OF_REAR_TIRES_APV"
  Divide2/1 -> Unit Delay3/1
  Constant5/1 -> Product2/3, Divide2/2  "GLB_NUMBER_OF_TRAILER_TIRES_APV"
  Constant/1 -> 2D_Lookup_Table/1  "GLB_STEER_TREAD_APV"
  Constant1/1 -> Divide/2, Product/3  "GLB_NUMBER_OF_FRONT_TIRES_APV"
  Constant2/1 -> 2D_Lookup_Table1/1  "GLB_DRIVE_TREAD_APV"
  Unit Delay2/1 -> 2D_Lookup_Table1/2

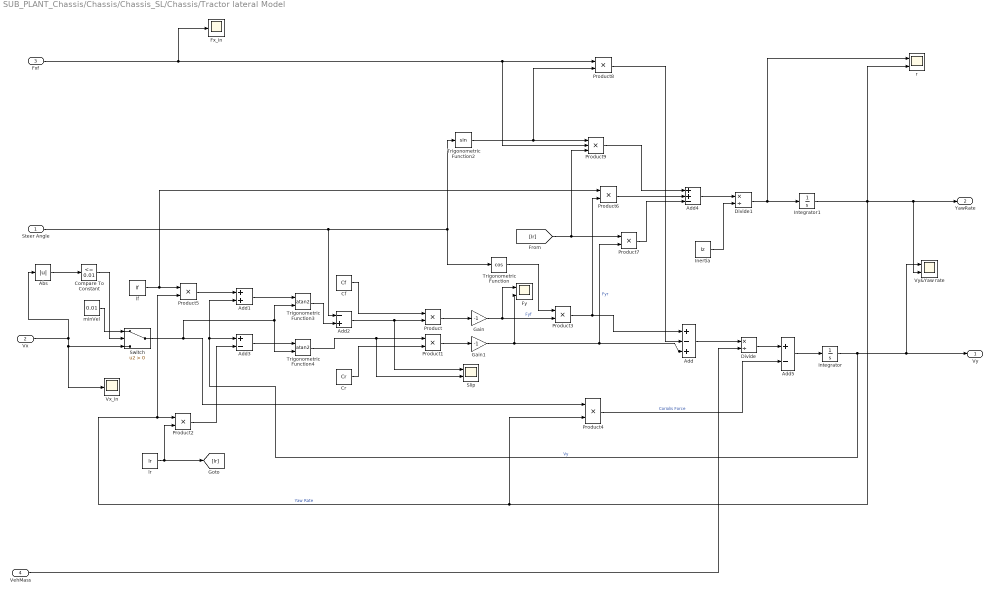
== system SUB_PLANT_Chassis/Chassis/Chassis_SL/Chassis/Tractor lateral Model ==
  Steer Angle : Inport
  Vx : Inport  Port=2
  Fxf : Inport  Port=3
  VehMass : Inport  Port=4
  Abs : Abs
  Add : Sum  Inputs=+-+
  Add1 : Sum
  Add2 : Sum  Inputs=-+
  Add3 : Sum  Inputs=+-
  Add4 : Sum  Inputs=++-
  Add5 : Sum  Inputs=+-
  Cf : Constant  Value=Cf
  Compare To Constant : simulink/Logic and Bit Operations/Compare To Constant  relop=<=  const=0.01  OutDataTypeStr=boolean
  Cr : Constant  Value=Cr
  Divide : Product  Inputs=*/
  Divide1 : Product  Inputs=*/
  Fx_in : Scope
  Fy : Scope  NumInputPorts=2
  Gain : Gain  Gain=-1
  Gain1 : Gain  Gain=-1
  Inertia : Constant  Value=Iz
  Integrator : Integrator
  Integrator1 : Integrator
  Product{,1..8} (9 alike) : Product
  Product9 : Product  Inputs=3
  Slip : Scope  NumInputPorts=2
  Switch : Switch  Criteria=u2 > Threshold
  Trigonometric Function : Trigonometry  Operator=cos
  Trigonometric Function2 : Trigonometry
  Trigonometric Function3 : Trigonometry  Operator=atan2
  Trigonometric Function4 : Trigonometry  Operator=atan2
  Vx_in : Scope
  Vy&Yaw rate : Scope  NumInputPorts=2
  lf : Constant  Value=lf
  lr : Constant  Value=lr
  minVel : Constant  Value=0.01
  r : Scope  NumInputPorts=2
  Vy : Outport
  YawRate : Outport  Port=2
  wires:
  minVel/1 -> Switch/1
  Switch/1 -> Product4/1, Trigonometric Function3/2, Trigonometric Function4/2
  Compare To Constant/1 -> Switch/2
  Abs/1 -> Compare To Constant/1
  VehMass/1 -> Divide/2
  Trigonometric Function2/1 -> Product9/1, Product8/2
  lr/1 -> [lr], Product2/2
  Integrator1/1 -> Product4/2, Product5/2, Product2/1, r/2, YawRate/1, Vy&Yaw rate/2  "Yaw Rate"
  Product6/1 -> Add4/2
  Product8/1 -> Add/2
  Vx/1 -> Abs/1, Switch/3, Vx_in/1
  Add4/1 -> Divide1/1
  Gain1/1 -> Add/3, Product7/2, Fy/2  "Fyr"
  Gain/1 -> Product3/2, Fy/1  "Fyf"
  Product3/1 -> Product6/2, Add/1
  Integrator/1 -> Vy&Yaw rate/1, Vy/1, Add1/2, Add3/1  "Vy"
  Product9/1 -> Add4/1
  [lr] -> Product9/3, Product7/1
  Fxf/1 -> Product9/2, Product8/1, Fx_in/1
  Inertia/1 -> Divide1/2
  Cr/1 -> Product1/2
  Product/1 -> Gain/1
  lf/1 -> Product6/1, Product5/1
  Cf/1 -> Product/1
  Divide1/1 -> r/1, Integrator1/1
  Product5/1 -> Add1/1
  Add3/1 -> Trigonometric Function4/1
  Steer Angle/1 -> Add2/1, Trigonometric Function/1, Trigonometric Function2/1
  Product7/1 -> Add4/3
  Add/1 -> Divide/1
  Product1/1 -> Gain1/1
  Add1/1 -> Trigonometric Function3/1
  Product2/1 -> Add3/2
  Trigonometric Function/1 -> Product3/1
  Add2/1 -> Slip/1, Product/2
  Trigonometric Function4/1 -> Slip/2, Product1/1
  Trigonometric Function3/1 -> Add2/2
  Add5/1 -> Integrator/1
  Divide/1 -> Add5/1
  Product4/1 -> Add5/2  "Coriolis Force"

== system SUB_PLANT_Chassis/Chassis/Chassis_SL/Chassis/Trailer Model ==
  Vx : Inport
  heading : Inport  Port=2
  Divide : Product  Inputs=**/
  IC : InitialCondition  Value=0
  Sum2 : Sum  Inputs=|+-
  Trailer Heading : Integrator  InitialCondition=heading_0  UpperSaturationLimit=pi  LowerSaturationLimit=-pi  WrapState=on
  Trailer Length : Constant  Value=15
  Trigonometric Function : Trigonometry
  wrap to pi1 : MATLAB Function  TreatAsAtomicUnit=on
  hitch angle : Outport
  wires:
  Trigonometric Function/1 -> Divide/1
  Sum2/1 -> wrap to pi1/1(u)
  heading/1 -> Sum2/1
  Trailer Length/1 -> Divide/3
  Trailer Heading/1 -> Sum2/2
  Divide/1 -> Trailer Heading/1
  wrap to pi1/1(y) -> IC/1, Trigonometric Function/1  "hitch angle"
  Vx/1 -> Divide/2
  IC/1 -> hitch angle/1

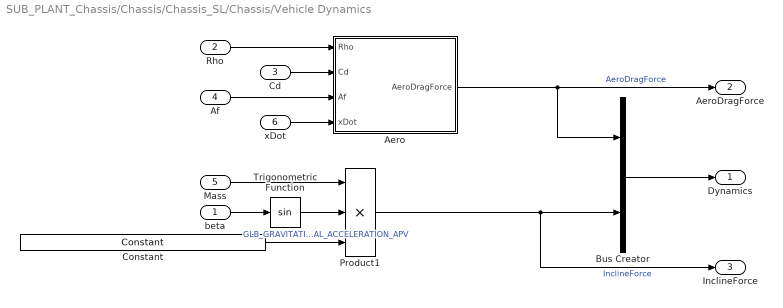
== system SUB_PLANT_Chassis/Chassis/Chassis_SL/Chassis/Vehicle Dynamics ==
  beta : Inport
  Rho : Inport  Port=2
  Cd : Inport  Port=3
  Af : Inport  Port=4
  Mass : Inport  Port=5
  xDot : Inport  Port=6
  Aero : Subsystem
  Bus Creator : BusCreator  Inputs=2
  Constant : PTC_MBDS_LIB/Extras/Sources/Constant  Value2=GLB_GRAVITATIONAL_ACCELERATION_APV  PTC_MBDS_BlockVersion=5.41  PTC_BlockType=PTC_MBDS_Constant
      settings: SourceProductName=PACCAR Technical Center MBDS Library
      settings: AttributesFormatString=|
      | Value: 9.80665016174
      | Unit: 'm/s^2'
  Product1 : Product  Inputs=3  RndMeth=Zero
  Trigonometric Function : Trigonometry
  Dynamics : Outport
  AeroDragForce : Outport  Port=2
  InclineForce : Outport  Port=3
  wires:
  Bus Creator/1 -> Dynamics/1
  beta/1 -> Trigonometric Function/1
  Product1/1 -> Bus Creator/2, InclineForce/1  "InclineForce"
  Mass/1 -> Product1/1
  Trigonometric Function/1 -> Product1/2
  Rho/1 -> Aero/1(Rho)
  Cd/1 -> Aero/2(Cd)
  Af/1 -> Aero/3(Af)
  Aero/1(AeroDragForce) -> AeroDragForce/1, Bus Creator/1  "AeroDragForce"
  xDot/1 -> Aero/4(xDot)
  Constant/1 -> Product1/3  "GLB_GRAVITATIONAL_ACCELERATION_APV"

== system SUB_PLANT_Chassis/Chassis/Chassis_SL/DriveAxleLosses/Divide_gtz ==
  num : Inport
  den : Inport  Port=2
  Enable : EnablePort
  Divide : Product  Inputs=*/
  out : Outport  OutputWhenDisabled=reset  InitialOutput=0
  wires:
  Divide/1 -> out/1
  num/1 -> Divide/1
  den/1 -> Divide/2
